simulink model "Practica_5_4"  (R2025b)
settings: Solver=VariableStepAuto  StartTime=0.0  StopTime=10.0  RelTol=1e-3
libraries: slpidlib x2
settings DebuggingCC: StateNameClashWarn=warning

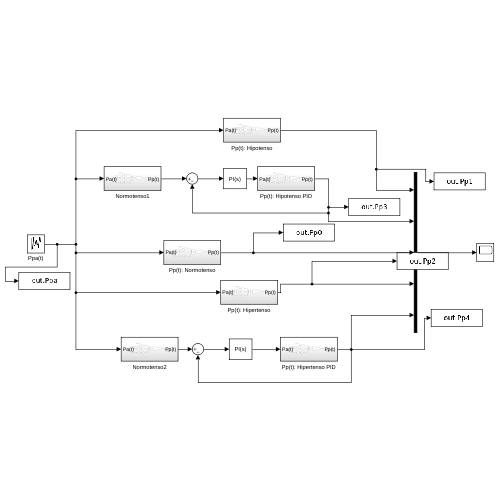
[thumbnail: Simulink's stored preview of the top-level diagram]
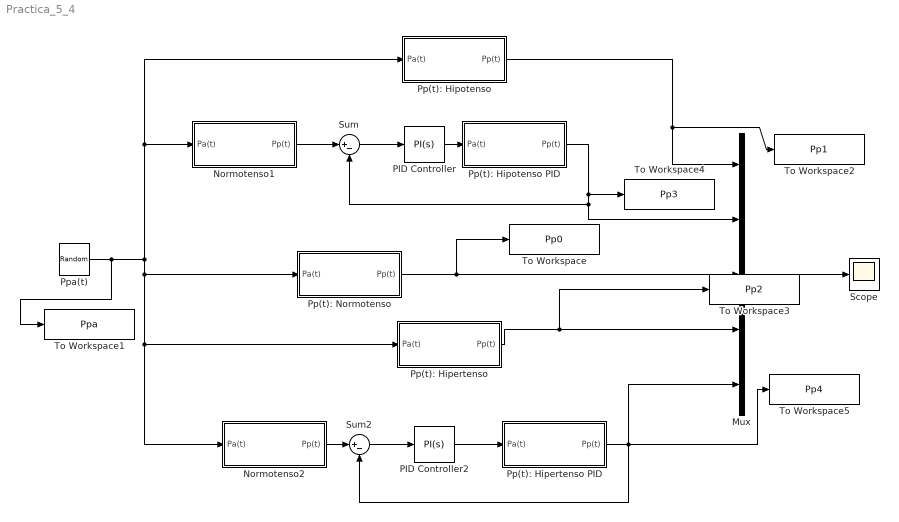
== system Practica_5_4 ==
  Mux : Mux  Inputs=5
  Normotenso1 : Subsystem
  Normotenso2 : Subsystem
  PID Controller : slpidlib/PID Controller  Controller=PI  Form=Parallel  TimeDomain=Continuous-time  UseExternalTs=off  SampleTime=-1  IntegratorMethod=Forward Euler  FilterMethod=Forward Euler  ControllerParametersSource=internal  P=4.2164E-05  I=3267.6867  UseKiTs=off  D=0  UseExternalDerivativeSource=off  N=100  UseFilter=on  TunerSelectOption=Transfer Function Based (PID Tuner App)  InitialConditionSource=internal  InitialConditionForIntegrator=0  InitialConditionForFilter=0  DifferentiatorICPrevScaledInput=0  ExternalReset=none  TrackingMode=off  Kt=1  LimitOutput=off  SatLimitsSource=internal  UpperSaturationLimit=inf  LowerSaturationLimit=-inf  LinearizeAsGain=on  AntiWindupMode=none  Kb=1  LimitIntegrator=off  UpperIntegratorSaturationLimit=inf  LowerIntegratorSaturationLimit=-inf  POutMin=[]  POutMax=[]  IOutMin=[]  IOutMax=[]  DOutMin=[]  DOutMax=[]  NOutMin=[]  NOutMax=[]  SumOutMin=[]  SumOutMax=[]  SaturationOutMin=[]  SaturationOutMax=[]  PParamMin=[]  PParamMax=[]  IParamMin=[]  IParamMax=[]  DParamMin=[]  DParamMax=[]  NParamMin=[]  NParamMax=[]  KbParamMin=[]  KbParamMax=[]  KtParamMin=[]  KtParamMax=[]  KbOutMin=[]  KbOutMax=[]  KtOutMin=[]  KtOutMax=[]  IntegratorOutMin=[]  IntegratorOutMax=[]  FilterOutMin=[]  FilterOutMax=[]  SumI1OutMin=[]  SumI1OutMax=[]  SumI2OutMin=[]  SumI2OutMax=[]  SumI3OutMin=[]  SumI3OutMax=[]  SumI4OutMin=[]  SumI4OutMax=[]  SumDOutMin=[]  SumDOutMax=[]  DifferentiatorOutMin=[]  DifferentiatorOutMax=[]  FilterDiffOutCoefMin=[]  FilterDiffOutCoefMax=[]  ReciprocalOutMin=[]  ReciprocalOutMax=[]  SumDenOutMin=[]  SumDenOutMax=[]  SumNumOutMin=[]  SumNumOutMax=[]  DivideOutMin=[]  DivideOutMax=[]  UdiffTsProdOutMin=[]  UdiffTsProdOutMax=[]  NTsProdOutMin=[]  NTsProdOutMax=[]  UintegralTsProdOutMin=[]  UintegralTsProdOutMax=[]  UngainTsProdOutMin=[]  UngainTsProdOutMax=[]  ClampingZeroOutDataTypeStr=Inherit: Inherit via back propagation  ClampingZeroOutMin=[]  ClampingZeroOutMax=[]  FilterDenConstantOutDataTypeStr=Inherit: Inherit via back propagation  FilterDenConstantOutMin=[]  FilterDenConstantOutMax=[]  PCopyOutDataTypeStr=Inherit: Inherit via back propagation  PCopyOutMin=[]  PCopyOutMax=[]  NCopyOutDataTypeStr=Inherit: Inherit via back propagation  NCopyOutMin=[]  NCopyOutMax=[]  IntegratorContinuousStateAttributes=''  IntegratorStateMustResolveToSignalObject=off  IntegratorRTWStateStorageClass=Auto  FilterContinuousStateAttributes=''  FilterStateMustResolveToSignalObject=off  FilterRTWStateStorageClass=Auto  ParallelPVariant=InternalParameters  IdealPVariant=Disabled  IVariant=InternalParameters  DVariant=Disabled  IntegratorVariant=Continuous  SatVariant=Disabled  AWVariant=Passthrough  PCopyVariant=Disabled  TRVariant=Disabled  FdbkBlocksVariant=Forward  IdealPFdbkVariant=Disabled  SatFdbkVariant=Disabled  DerivativeFilterVariant=Disabled  NVariant=Disabled  NCopyVariant=Disabled_SignalSpec  FilterICVariant=Disabled  IntegratorICVariant=InternalICs  ExternalResetVariant=Disabled  TRSumVariant=Passthrough  SumFdbkVariant=Disabled  SumVariant=Sum_PI  TsampFilterVariant=InternalTs  TsampNgainVariant=Passthrough  TsampIntegralVariant=Disabled_SignalSpec  ExternalSaturationOutDataTypeStr=Inherit: Same as second input  DerivativeSourceVariant=Disabled  PreIntVariant=InternalPreInt
  PID Controller2 : slpidlib/PID Controller  Controller=PI  Form=Parallel  TimeDomain=Continuous-time  UseExternalTs=off  SampleTime=-1  IntegratorMethod=Forward Euler  FilterMethod=Forward Euler  ControllerParametersSource=internal  P=10  I=3275.21611480  UseKiTs=off  D=0  UseExternalDerivativeSource=off  N=100  UseFilter=on  TunerSelectOption=Transfer Function Based (PID Tuner App)  InitialConditionSource=internal  InitialConditionForIntegrator=0  InitialConditionForFilter=0  DifferentiatorICPrevScaledInput=0  ExternalReset=none  TrackingMode=off  Kt=1  LimitOutput=off  SatLimitsSource=internal  UpperSaturationLimit=inf  LowerSaturationLimit=-inf  LinearizeAsGain=on  AntiWindupMode=none  Kb=1  LimitIntegrator=off  UpperIntegratorSaturationLimit=inf  LowerIntegratorSaturationLimit=-inf  POutMin=[]  POutMax=[]  IOutMin=[]  IOutMax=[]  DOutMin=[]  DOutMax=[]  NOutMin=[]  NOutMax=[]  SumOutMin=[]  SumOutMax=[]  SaturationOutMin=[]  SaturationOutMax=[]  PParamMin=[]  PParamMax=[]  IParamMin=[]  IParamMax=[]  DParamMin=[]  DParamMax=[]  NParamMin=[]  NParamMax=[]  KbParamMin=[]  KbParamMax=[]  KtParamMin=[]  KtParamMax=[]  KbOutMin=[]  KbOutMax=[]  KtOutMin=[]  KtOutMax=[]  IntegratorOutMin=[]  IntegratorOutMax=[]  FilterOutMin=[]  FilterOutMax=[]  SumI1OutMin=[]  SumI1OutMax=[]  SumI2OutMin=[]  SumI2OutMax=[]  SumI3OutMin=[]  SumI3OutMax=[]  SumI4OutMin=[]  SumI4OutMax=[]  SumDOutMin=[]  SumDOutMax=[]  DifferentiatorOutMin=[]  DifferentiatorOutMax=[]  FilterDiffOutCoefMin=[]  FilterDiffOutCoefMax=[]  ReciprocalOutMin=[]  ReciprocalOutMax=[]  SumDenOutMin=[]  SumDenOutMax=[]  SumNumOutMin=[]  SumNumOutMax=[]  DivideOutMin=[]  DivideOutMax=[]  UdiffTsProdOutMin=[]  UdiffTsProdOutMax=[]  NTsProdOutMin=[]  NTsProdOutMax=[]  UintegralTsProdOutMin=[]  UintegralTsProdOutMax=[]  UngainTsProdOutMin=[]  UngainTsProdOutMax=[]  ClampingZeroOutDataTypeStr=Inherit: Inherit via back propagation  ClampingZeroOutMin=[]  ClampingZeroOutMax=[]  FilterDenConstantOutDataTypeStr=Inherit: Inherit via back propagation  FilterDenConstantOutMin=[]  FilterDenConstantOutMax=[]  PCopyOutDataTypeStr=Inherit: Inherit via back propagation  PCopyOutMin=[]  PCopyOutMax=[]  NCopyOutDataTypeStr=Inherit: Inherit via back propagation  NCopyOutMin=[]  NCopyOutMax=[]  IntegratorContinuousStateAttributes=''  IntegratorStateMustResolveToSignalObject=off  IntegratorRTWStateStorageClass=Auto  FilterContinuousStateAttributes=''  FilterStateMustResolveToSignalObject=off  FilterRTWStateStorageClass=Auto  ParallelPVariant=InternalParameters  IdealPVariant=Disabled  IVariant=InternalParameters  DVariant=Disabled  IntegratorVariant=Continuous  SatVariant=Disabled  AWVariant=Passthrough  PCopyVariant=Disabled  TRVariant=Disabled  FdbkBlocksVariant=Forward  IdealPFdbkVariant=Disabled  SatFdbkVariant=Disabled  DerivativeFilterVariant=Disabled  NVariant=Disabled  NCopyVariant=Disabled_SignalSpec  FilterICVariant=Disabled  IntegratorICVariant=InternalICs  ExternalResetVariant=Disabled  TRSumVariant=Passthrough  SumFdbkVariant=Disabled  SumVariant=Sum_PI  TsampFilterVariant=InternalTs  TsampNgainVariant=Passthrough  TsampIntegralVariant=Disabled_SignalSpec  ExternalSaturationOutDataTypeStr=Inherit: Same as second input  DerivativeSourceVariant=Disabled  PreIntVariant=InternalPreInt
  Pp(t): Hipertenso : Subsystem
  Pp(t): Hipertenso PID : Subsystem
  Pp(t): Hipotenso : Subsystem
  Pp(t): Hipotenso PID : Subsystem
  Pp(t): Normotenso : Subsystem
  Ppa(t) : UniformRandomNumber  Minimum=-0.2  Seed=106  SampleTime=0.5
  Scope : Scope
      settings: ActiveDisplayYMinimum=-0.27073049295196561  ActiveDisplayYMaximum=1.1774972981597891
  Sum : Sum  Inputs=|+-
  Sum2 : Sum  Inputs=|+-
  To Workspace : ToWorkspace  VariableName=Pp0  SampleTime=-1
  To Workspace1 : ToWorkspace  VariableName=Ppa  SampleTime=-1
  To Workspace2 : ToWorkspace  VariableName=Pp1  SampleTime=-1
  To Workspace3 : ToWorkspace  VariableName=Pp2  SampleTime=-1
  To Workspace4 : ToWorkspace  VariableName=Pp3  SampleTime=-1
  To Workspace5 : ToWorkspace  VariableName=Pp4  SampleTime=-1
  wires:
  Ppa(t)/1 -> To Workspace1/1, Normotenso2/1(Pa(t)), Pp(t): Hipertenso/1(Pa(t)), Pp(t): Normotenso/1(Pa(t)), Pp(t): Hipotenso/1(Pa(t)), Normotenso1/1(Pa(t))
  Pp(t): Hipotenso/1(Pp(t)) -> To Workspace2/1, Mux/1
  Mux/1 -> Scope/1
  PID Controller/1 -> Pp(t): Hipotenso PID/1(Pa(t))
  Normotenso1/1(Pp(t)) -> Sum/1
  Sum/1 -> PID Controller/1
  Pp(t): Hipotenso PID/1(Pp(t)) -> Sum/2, Mux/2, To Workspace4/1
  Pp(t): Normotenso/1(Pp(t)) -> To Workspace/1, Mux/3
  Normotenso2/1(Pp(t)) -> Sum2/1
  Sum2/1 -> PID Controller2/1
  PID Controller2/1 -> Pp(t): Hipertenso PID/1(Pa(t))
  Pp(t): Hipertenso/1(Pp(t)) -> To Workspace3/1, Mux/4
  Pp(t): Hipertenso PID/1(Pp(t)) -> To Workspace5/1, Mux/5, Sum2/2

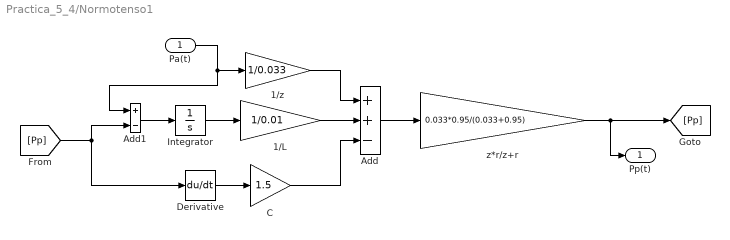
== system Practica_5_4/Normotenso1 ==
  Pa(t) : Inport
  1/L : Gain  Gain=1/0.01
  1/z : Gain  Gain=1/0.033
  Add : Sum  Inputs=++-
  Add1 : Sum  Inputs=+-
  C : Gain  Gain=1.5
  Derivative : Derivative
  Integrator : Integrator
  z*r/z+r : Gain  Gain=0.033*0.95/(0.033+0.95)
  Pp(t) : Outport
  wires:
  1/z/1 -> Add/1
  1/L/1 -> Add/2
  C/1 -> Add/3
  Derivative/1 -> C/1
  Integrator/1 -> 1/L/1
  Pa(t)/1 -> Add1/1, 1/z/1
  Add1/1 -> Integrator/1
  Add/1 -> z*r/z+r/1
  z*r/z+r/1 -> [Pp], Pp(t)/1
  [Pp] -> Derivative/1, Add1/2

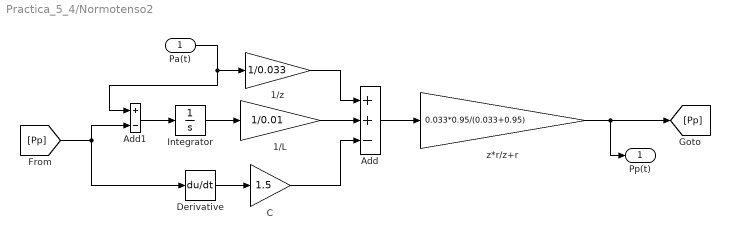
== system Practica_5_4/Normotenso2 ==
  Pa(t) : Inport
  1/L : Gain  Gain=1/0.01
  1/z : Gain  Gain=1/0.033
  Add : Sum  Inputs=++-
  Add1 : Sum  Inputs=+-
  C : Gain  Gain=1.5
  Derivative : Derivative
  Integrator : Integrator
  z*r/z+r : Gain  Gain=0.033*0.95/(0.033+0.95)
  Pp(t) : Outport
  wires:
  1/z/1 -> Add/1
  1/L/1 -> Add/2
  C/1 -> Add/3
  Derivative/1 -> C/1
  Integrator/1 -> 1/L/1
  Pa(t)/1 -> Add1/1, 1/z/1
  Add1/1 -> Integrator/1
  Add/1 -> z*r/z+r/1
  z*r/z+r/1 -> [Pp], Pp(t)/1
  [Pp] -> Derivative/1, Add1/2

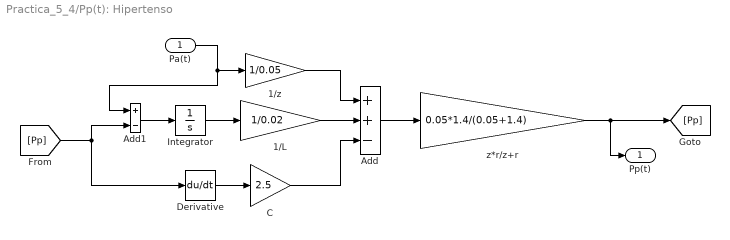
== system Practica_5_4/Pp(t): Hipertenso ==
  Pa(t) : Inport
  1/L : Gain  Gain=1/0.02
  1/z : Gain  Gain=1/0.05
  Add : Sum  Inputs=++-
  Add1 : Sum  Inputs=+-
  C : Gain  Gain=2.5
  Derivative : Derivative
  Integrator : Integrator
  z*r/z+r : Gain  Gain=0.05*1.4/(0.05+1.4)
  Pp(t) : Outport
  wires:
  1/z/1 -> Add/1
  1/L/1 -> Add/2
  C/1 -> Add/3
  Derivative/1 -> C/1
  Integrator/1 -> 1/L/1
  Pa(t)/1 -> Add1/1, 1/z/1
  Add1/1 -> Integrator/1
  Add/1 -> z*r/z+r/1
  z*r/z+r/1 -> [Pp], Pp(t)/1
  [Pp] -> Derivative/1, Add1/2

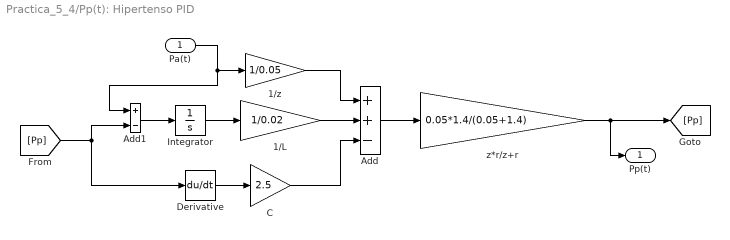
== system Practica_5_4/Pp(t): Hipertenso PID ==
  Pa(t) : Inport
  1/L : Gain  Gain=1/0.02
  1/z : Gain  Gain=1/0.05
  Add : Sum  Inputs=++-
  Add1 : Sum  Inputs=+-
  C : Gain  Gain=2.5
  Derivative : Derivative
  Integrator : Integrator
  z*r/z+r : Gain  Gain=0.05*1.4/(0.05+1.4)
  Pp(t) : Outport
  wires:
  1/z/1 -> Add/1
  1/L/1 -> Add/2
  C/1 -> Add/3
  Derivative/1 -> C/1
  Integrator/1 -> 1/L/1
  Pa(t)/1 -> Add1/1, 1/z/1
  Add1/1 -> Integrator/1
  Add/1 -> z*r/z+r/1
  z*r/z+r/1 -> [Pp], Pp(t)/1
  [Pp] -> Derivative/1, Add1/2

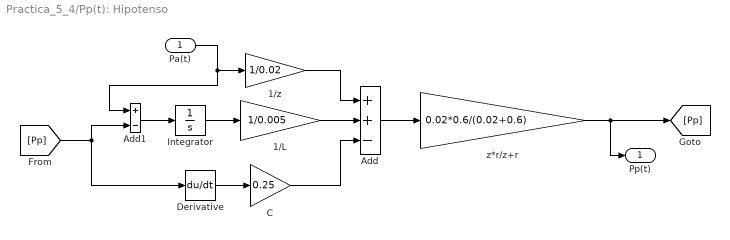
== system Practica_5_4/Pp(t): Hipotenso ==
  Pa(t) : Inport
  1/L : Gain  Gain=1/0.005
  1/z : Gain  Gain=1/0.02
  Add : Sum  Inputs=++-
  Add1 : Sum  Inputs=+-
  C : Gain  Gain=0.25
  Derivative : Derivative
  Integrator : Integrator
  z*r/z+r : Gain  Gain=0.02*0.6/(0.02+0.6)
  Pp(t) : Outport
  wires:
  1/z/1 -> Add/1
  1/L/1 -> Add/2
  C/1 -> Add/3
  Derivative/1 -> C/1
  Integrator/1 -> 1/L/1
  Pa(t)/1 -> Add1/1, 1/z/1
  Add1/1 -> Integrator/1
  Add/1 -> z*r/z+r/1
  z*r/z+r/1 -> [Pp], Pp(t)/1
  [Pp] -> Derivative/1, Add1/2

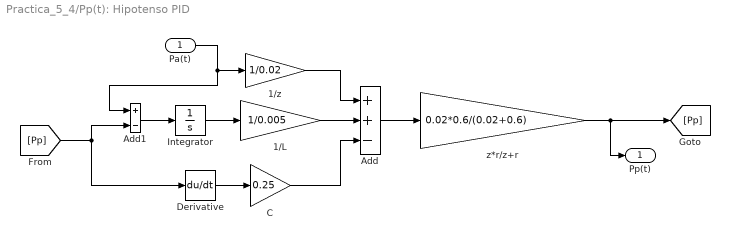
== system Practica_5_4/Pp(t): Hipotenso PID ==
  Pa(t) : Inport
  1/L : Gain  Gain=1/0.005
  1/z : Gain  Gain=1/0.02
  Add : Sum  Inputs=++-
  Add1 : Sum  Inputs=+-
  C : Gain  Gain=0.25
  Derivative : Derivative
  Integrator : Integrator
  z*r/z+r : Gain  Gain=0.02*0.6/(0.02+0.6)
  Pp(t) : Outport
  wires:
  1/z/1 -> Add/1
  1/L/1 -> Add/2
  C/1 -> Add/3
  Derivative/1 -> C/1
  Integrator/1 -> 1/L/1
  Pa(t)/1 -> Add1/1, 1/z/1
  Add1/1 -> Integrator/1
  Add/1 -> z*r/z+r/1
  z*r/z+r/1 -> [Pp], Pp(t)/1
  [Pp] -> Derivative/1, Add1/2

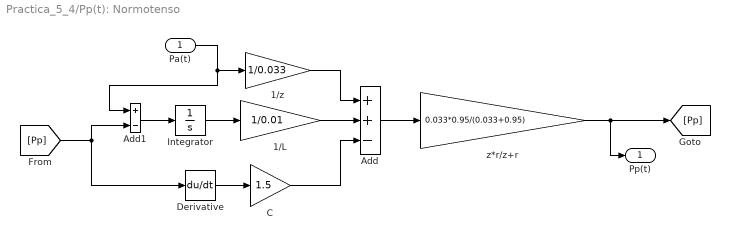
== system Practica_5_4/Pp(t): Normotenso ==
  Pa(t) : Inport
  1/L : Gain  Gain=1/0.01
  1/z : Gain  Gain=1/0.033
  Add : Sum  Inputs=++-
  Add1 : Sum  Inputs=+-
  C : Gain  Gain=1.5
  Derivative : Derivative
  Integrator : Integrator
  z*r/z+r : Gain  Gain=0.033*0.95/(0.033+0.95)
  Pp(t) : Outport
  wires:
  1/z/1 -> Add/1
  1/L/1 -> Add/2
  C/1 -> Add/3
  Derivative/1 -> C/1
  Integrator/1 -> 1/L/1
  Pa(t)/1 -> Add1/1, 1/z/1
  Add1/1 -> Integrator/1
  Add/1 -> z*r/z+r/1
  z*r/z+r/1 -> [Pp], Pp(t)/1
  [Pp] -> Derivative/1, Add1/2
